simulink model "FRDMKL25Z"  (R2016b)
settings: Solver=FixedStepDiscrete  StartTime=0.0  StopTime=10.0  RelTol=1e-3  EnableMultiTasking=on
undefined symbols (not defined in the file): D5, PTA5
libraries: frdmkl25zlib x4
settings Model: ExtModeTrigDuration=5  Creator=admin  LastModifiedBy=admin
settings OptimizationCC: MaxStackSize=64
settings DebuggingCC: ParameterTunabilityLossMsg=error
settings HardwareCC: ProdBitPerPointer=32  ProdBitPerSizeT=32  ProdBitPerPtrDiffT=32  ProdLargestAtomicInteger=Long  ProdLargestAtomicFloat=Double  ProdWordSize=32  ProdHWDeviceType=ARM Compatible->ARM Cortex
settings RTWCC: SystemTargetFile=ert.tlc  HardwareBoard=NXP FRDM-KL25Z  TLCOptions=-aInlineSetEventsForThisBaseRateFcn=TLC_FALSE -aSuppressMultiTaskScheduler=TLC_FALSE -aRateBasedStepFcn=1  TemplateMakefile=ert_default_tmf  Description=Embedded Coder  GenerateReport=on  Toolchain=GNU Tools for ARM Embedded Processors  IncludeHyperlinkInReport=on  LaunchReport=on  GenerateTraceInfo=on  GenerateTraceReport=on  GenerateTraceReportSl=on  GenerateTraceReportSf=on  GenerateTraceReportEml=on
settings CodeAppCC: ForceParamTrailComments=on  IgnoreCustomStorageClasses=off  OperatorAnnotations=on  SimulinkDataObjDesc=on  SFDataObjDesc=on  MATLABFcnDesc=on  InsertBlockDesc=on  MATLABSourceComments=on

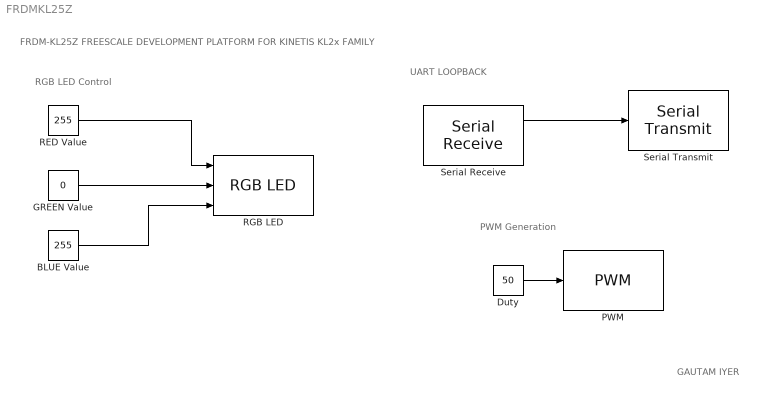
== system FRDMKL25Z ==
  note: FRDM-KL25Z FREESCALE DEVELOPMENT PLATFORM FOR KINETIS KL2x FAMILY
  note: UART LOOPBACK
  note: PWM Generation
  note: RGB LED Control
  note: GAUTAM IYER
  BLUE Value : Constant  Value=255  SampleTime=1
  Duty : Constant  Value=50
  GREEN Value : Constant  Value=0  SampleTime=1
  PWM : frdmkl25zlib/PWM  WhichPin=PTA5 (D5)  WhichTimer=TPM0  InitialDutyCycle=0
  RED Value : Constant  Value=255  OutDataTypeStr=uint8  SampleTime=1
  RGB LED : frdmkl25zlib/RGB LED
  Serial Receive : frdmkl25zlib/Serial Receive  uart=UART0  DataType=int8  DataLength=1  SampleTime=0.1
  Serial Transmit : frdmkl25zlib/Serial Transmit  uart=UART0  sendmode=putc
  wires:
  Serial Receive/1 -> Serial Transmit/1
  Duty/1 -> PWM/1
  BLUE Value/1 -> RGB LED/3
  GREEN Value/1 -> RGB LED/2
  RED Value/1 -> RGB LED/1
